simulink model "regen"  (R2024b)
settings: Solver=VariableStepAuto  StartTime=0.0  StopTime=10  RelTol=1e-3
libraries: fuzblock x1
settings Model: Creator=jessi  LastModifiedBy=Aditya

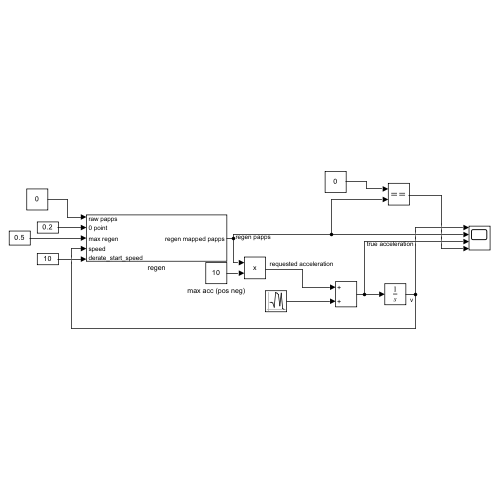
[thumbnail: Simulink's stored preview of the top-level diagram]
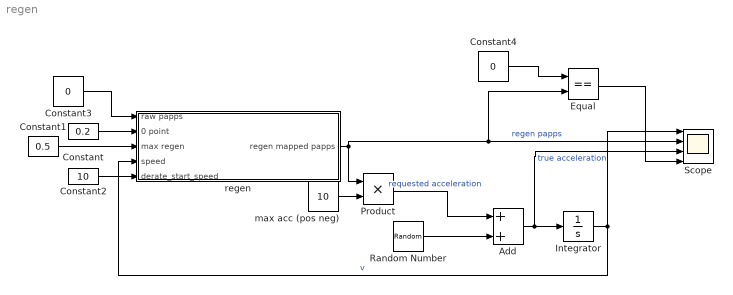
== system regen ==
  Add : Sum
  Constant : Constant  Value=0.2
  Constant1 : Constant  Value=0.5
  Constant2 : Constant  Value=10
  Constant3 : Constant  Value=0
  Constant4 : Constant  Value=0
  Equal : RelationalOperator  Operator===  OutDataTypeStr=boolean  RndMeth=Simplest  InputSameDT=off
  Integrator : Integrator  InitialCondition=20
  Product : Product
  Random Number : RandomNumber  Variance=2  SampleTime=0.01
  Scope : Scope  NumInputPorts=4
  max acc (pos neg) : Constant  Value=10
  regen : Subsystem
  wires:
  regen/1(regen mapped papps) -> Equal/2, Scope/2, Product/1  "regen papps"
  Constant/1 -> regen/2(0 point)
  Constant1/1 -> regen/3(max regen)
  Constant2/1 -> regen/5(derate_start_speed)
  Product/1 -> Add/1  "requested acceleration"
  Integrator/1 -> Scope/1, regen/4(speed)  "v"
  max acc (pos neg)/1 -> Product/2
  Constant3/1 -> regen/1(raw papps)
  Random Number/1 -> Add/2
  Add/1 -> Integrator/1, Scope/3  "true acceleration"
  Constant4/1 -> Equal/1
  Equal/1 -> Scope/4

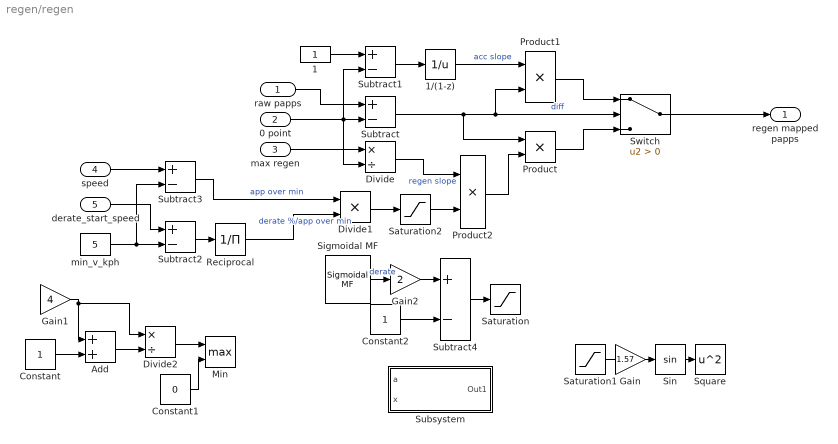
== system regen/regen ==
  raw papps : Inport
  0 point : Inport  Port=2
  max regen : Inport  Port=3
  speed : Inport  Port=4
  derate_start_speed : Inport  Port=5
  1 : Constant
  1/(1-z) : Math  Operator=reciprocal  SignedPower=on
  Add : Sum
  Constant : Constant
  Constant1 : Constant  Value=0
  Constant2 : Constant
  Divide : Product  Inputs=*/
  Divide1 : Product  Inputs=**
  Divide2 : Product  Inputs=*/
  Gain : Gain  Gain=1.57
  Gain1 : Gain  Gain=4
  Gain2 : Gain  Gain=2
  Min : MinMax  Function=max  Inputs=2
  Product : Product
  Product1 : Product
  Product2 : Product
  Reciprocal : Product  Inputs=/
  Saturation : Saturate  UpperLimit=1  LowerLimit=0
  Saturation1 : Saturate  UpperLimit=1  LowerLimit=0
  Saturation2 : Saturate  UpperLimit=1  LowerLimit=0
  Sigmoidal MF : fuzblock/Membership  Functions/Sigmoidal MF  a=5.5  c=6/10+0.6/10
  Sin : Trigonometry
  Square : Math  Operator=square
  Subsystem : Subsystem
  Subtract{,1..4} (5 alike) : Sum  Inputs=+-
  Switch : Switch  Criteria=u2 > Threshold  SaturateOnIntegerOverflow=off  InputSameDT=off
  min_v_kph : Constant  Value=5
  regen mapped papps : Outport
  wires:
  1/1 -> Subtract1/1
  Subtract/1 -> Switch/2, Product1/2, Product/1  "diff"
  0 point/1 -> Divide/2, Subtract/2, Subtract1/2
  Product/1 -> Switch/3
  Subtract1/1 -> 1/(1-z)/1
  1/(1-z)/1 -> Product1/1  "acc slope"
  Product1/1 -> Switch/1
  Switch/1 -> regen mapped papps/1
  max regen/1 -> Divide/1
  raw papps/1 -> Subtract/1
  Divide/1 -> Product2/1  "regen slope"
  derate_start_speed/1 -> Subtract2/1
  Subtract2/1 -> Reciprocal/1
  min_v_kph/1 -> Subtract2/2, Subtract3/2
  speed/1 -> Subtract3/1
  Subtract3/1 -> Divide1/1  "app over min"
  Product2/1 -> Product/2
  Reciprocal/1 -> Divide1/2  "derate %/app over min"
  Sin/1 -> Square/1
  Saturation1/1 -> Sin/1
  Gain1/1 -> Divide2/1, Add/1
  Constant/1 -> Add/2
  Add/1 -> Divide2/2
  Divide2/1 -> Min/1
  Constant1/1 -> Min/2
  Sigmoidal MF/1 -> Gain2/1  "derate"
  Constant2/1 -> Subtract4/2
  Gain2/1 -> Subtract4/1
  Subtract4/1 -> Saturation/1
  Divide1/1 -> Saturation2/1
  Saturation2/1 -> Product2/2

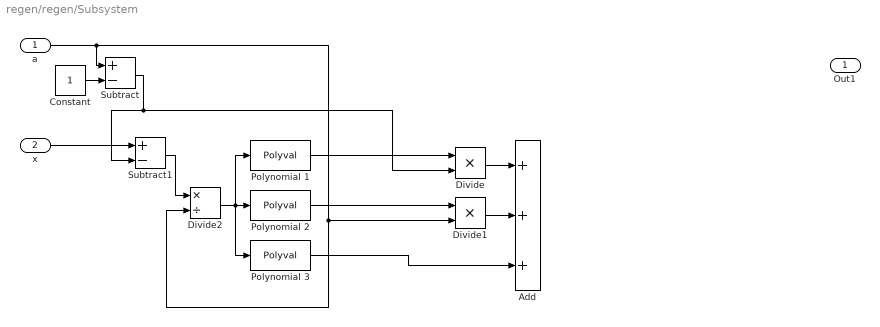
== system regen/regen/Subsystem ==
  a : Inport
  x : Inport  Port=2
  Add : Sum  Inputs=+++
  Constant : Constant
  Divide : Product  Inputs=**
  Divide1 : Product  Inputs=**
  Divide2 : Product  Inputs=*/
  Polynomial 1 : Polyval  Coefs=[2, -3, 0, 1]
  Polynomial 2 : Polyval  Coefs=[1, -2, 1, 0]
  Polynomial 3 : Polyval  Coefs=[-2, 3, 0, 0]
  Subtract : Sum  Inputs=+-
  Subtract1 : Sum  Inputs=+-
  Out1 : Outport
  wires:
  a/1 -> Divide2/2, Divide1/2, Subtract/1
  Polynomial 3/1 -> Add/3
  Polynomial 2/1 -> Divide1/1
  Polynomial 1/1 -> Divide/1
  Constant/1 -> Subtract/2
  Subtract/1 -> Subtract1/2, Divide/2
  Divide1/1 -> Add/2
  Divide/1 -> Add/1
  x/1 -> Subtract1/1
  Subtract1/1 -> Divide2/1
  Divide2/1 -> Polynomial 1/1, Polynomial 2/1, Polynomial 3/1
